simulink model "manul_model_stage15_complete"  (R2025a)
settings: Solver=ode3  StartTime=0.0  StopTime=0.3  FixedStep=Ts_power  RelTol=1e-3
InitFcn:
  | run('D:/PV_MPPT/PV_ESS_MPC_Manul_Reproduction/experiments/stage15_bus_stability_20260814/pvess_stage15_busfix_init.m')
values from neighbouring files (symbols this model uses):
  a_vbat_limit = exp(-2*pi*fc_vbat_limit*Ts_bat_ctrl)    [pvess_stage15_busfix_init.m]    (also in pvess_stage15_busfix_init_pre_cpl_20260817.m; pvess_stage15_busfix_init_pre_gridpi_tuning_20260817.m)
  Ad_mpvc = expm(A_mpvc*Ts_mpc)    [pvess_beginner_init_baseline.m]    (also in pvess_stage15_busfix_init.m; pvess_stage15_busfix_init_pre_cpl_20260817.m; pvess_stage15_busfix_init_pre_engineering_20260816.m; pvess_stage15_busfix_init_pre_gridpi_tuning_20260817.m)
  Bd_mpvc = A_mpvc\((Ad_mpvc-eye(2))*B_mpvc)    [pvess_beginner_init_baseline.m]    (also in pvess_stage15_busfix_init.m; pvess_stage15_busfix_init_pre_cpl_20260817.m; pvess_stage15_busfix_init_pre_engineering_20260816.m; pvess_stage15_busfix_init_pre_gridpi_tuning_20260817.m)
  Cdc = 18e-3    (= 0.018)    [pvess_beginner_init_baseline.m]    (also in pvess_stage15_busfix_init.m; pvess_stage15_busfix_init_pre_cpl_20260817.m; pvess_stage15_busfix_init_pre_engineering_20260816.m; pvess_stage15_busfix_init_pre_gridpi_tuning_20260817.m)
  Cpv = 10e-3    (= 0.01)    [pvess_beginner_init_baseline.m]    (also in pvess_stage15_busfix_init.m; pvess_stage15_busfix_init_pre_cpl_20260817.m; pvess_stage15_busfix_init_pre_engineering_20260816.m; pvess_stage15_busfix_init_pre_gridpi_tuning_20260817.m)
  Db0 = 1 - V_bat_nom/Vdc_ref    (= 0.75)    [pvess_beginner_init_baseline.m]    (also in pvess_stage15_busfix_init.m; pvess_stage15_busfix_init_pre_cpl_20260817.m; pvess_stage15_busfix_init_pre_engineering_20260816.m; pvess_stage15_busfix_init_pre_gridpi_tuning_20260817.m)
  Db_max = 0.95    [pvess_beginner_init_baseline.m]    (also in pvess_stage15_busfix_init.m; pvess_stage15_busfix_init_pre_cpl_20260817.m; pvess_stage15_busfix_init_pre_engineering_20260816.m; pvess_stage15_busfix_init_pre_gridpi_tuning_20260817.m)
  Db_min = 0.05    [pvess_beginner_init_baseline.m]    (also in pvess_stage15_busfix_init.m; pvess_stage15_busfix_init_pre_cpl_20260817.m; pvess_stage15_busfix_init_pre_engineering_20260816.m; pvess_stage15_busfix_init_pre_gridpi_tuning_20260817.m)
  Dcorr_max = Db_max - Db0    (= 0.2)    [pvess_stage15_busfix_init.m]    (also in pvess_stage15_busfix_init_pre_cpl_20260817.m; pvess_stage15_busfix_init_pre_gridpi_tuning_20260817.m)
  Dcorr_min = -0.25    [pvess_stage15_busfix_init.m]    (also in pvess_stage15_busfix_init_pre_cpl_20260817.m; pvess_stage15_busfix_init_pre_gridpi_tuning_20260817.m)
  Dpv0 = 1 - 547/Vdc_ref    (= 0.544166666667)    [pvess_beginner_init_baseline.m]    (also in pvess_stage15_busfix_init.m; pvess_stage15_busfix_init_pre_cpl_20260817.m; pvess_stage15_busfix_init_pre_engineering_20260816.m; pvess_stage15_busfix_init_pre_gridpi_tuning_20260817.m)
  Dpv_curtail_bias = 0.506    [pvess_stage15_busfix_init.m]    (also in pvess_stage15_busfix_init_pre_cpl_20260817.m; pvess_stage15_busfix_init_pre_engineering_20260816.m; pvess_stage15_busfix_init_pre_gridpi_tuning_20260817.m)
  Dpv_max = 0.75    [pvess_beginner_init_baseline.m]    (also in pvess_stage15_busfix_init.m; pvess_stage15_busfix_init_pre_cpl_20260817.m; pvess_stage15_busfix_init_pre_engineering_20260816.m; pvess_stage15_busfix_init_pre_gridpi_tuning_20260817.m)
  Dpv_min = 0.35    [pvess_beginner_init_baseline.m]    (also in pvess_stage15_busfix_init.m; pvess_stage15_busfix_init_pre_cpl_20260817.m; pvess_stage15_busfix_init_pre_engineering_20260816.m; pvess_stage15_busfix_init_pre_gridpi_tuning_20260817.m)
  Dpv_slew_down = -5.0    (= -5)    [pvess_stage15_busfix_init.m]    (also in pvess_stage15_busfix_init_pre_cpl_20260817.m; pvess_stage15_busfix_init_pre_engineering_20260816.m; pvess_stage15_busfix_init_pre_gridpi_tuning_20260817.m)
  Dpv_slew_up = 1.0    (= 1)    [pvess_stage15_busfix_init.m]    (also in pvess_stage15_busfix_init_pre_cpl_20260817.m; pvess_stage15_busfix_init_pre_engineering_20260816.m; pvess_stage15_busfix_init_pre_gridpi_tuning_20260817.m)
  Dpv_step = 2e-4    (= 0.0002)    [pvess_beginner_init_baseline.m]    (also in pvess_stage15_busfix_init.m; pvess_stage15_busfix_init_pre_cpl_20260817.m; pvess_stage15_busfix_init_pre_engineering_20260816.m; pvess_stage15_busfix_init_pre_gridpi_tuning_20260817.m)
  eps_dI = 1e-3    (= 0.001)    [pvess_beginner_init_baseline.m]    (also in pvess_stage15_busfix_init.m; pvess_stage15_busfix_init_pre_cpl_20260817.m; pvess_stage15_busfix_init_pre_engineering_20260816.m; pvess_stage15_busfix_init_pre_gridpi_tuning_20260817.m)
  eps_dV = 1e-3    (= 0.001)    [pvess_beginner_init_baseline.m]    (also in pvess_stage15_busfix_init.m; pvess_stage15_busfix_init_pre_cpl_20260817.m; pvess_stage15_busfix_init_pre_engineering_20260816.m; pvess_stage15_busfix_init_pre_gridpi_tuning_20260817.m)
  eps_inc = 1e-4    (= 0.0001)    [pvess_beginner_init_baseline.m]    (also in pvess_stage15_busfix_init.m; pvess_stage15_busfix_init_pre_cpl_20260817.m; pvess_stage15_busfix_init_pre_engineering_20260816.m; pvess_stage15_busfix_init_pre_gridpi_tuning_20260817.m)
  f_grid = 50    [pvess_beginner_init_baseline.m]    (also in pvess_stage15_busfix_init.m; pvess_stage15_busfix_init_pre_cpl_20260817.m; pvess_stage15_busfix_init_pre_engineering_20260816.m; pvess_stage15_busfix_init_pre_gridpi_tuning_20260817.m)
  freq_threshold = 0.15    [pvess_beginner_init_baseline.m]    (also in pvess_stage15_busfix_init.m; pvess_stage15_busfix_init_pre_cpl_20260817.m; pvess_stage15_busfix_init_pre_engineering_20260816.m; pvess_stage15_busfix_init_pre_gridpi_tuning_20260817.m)
  Iac_rated_lv = S_tr/(sqrt(3)*V_tr_lv)    [pvess_stage15_busfix_init.m]    (also in pvess_stage15_busfix_init_pre_cpl_20260817.m; pvess_stage15_busfix_init_pre_gridpi_tuning_20260817.m)
  Ibat_chg_hw = Ibat_max    (= 1666.66666667)    [pvess_stage15_busfix_init.m]    (also in pvess_stage15_busfix_init_pre_cpl_20260817.m; pvess_stage15_busfix_init_pre_gridpi_tuning_20260817.m)
  Ibat_curtail_release = -0.8*Ibat_max    (= -1333.33333333)    [pvess_stage15_busfix_init.m]    (also in pvess_stage15_busfix_init_pre_cpl_20260817.m; pvess_stage15_busfix_init_pre_engineering_20260816.m; pvess_stage15_busfix_init_pre_gridpi_tuning_20260817.m)
  Ibat_dis_hw = Ibat_max    (= 1666.66666667)    [pvess_stage15_busfix_init.m]    (also in pvess_stage15_busfix_init_pre_cpl_20260817.m; pvess_stage15_busfix_init_pre_gridpi_tuning_20260817.m)
  Ibat_max = P_bat_rated/V_bat_nom    (= 1666.66666667)    [pvess_beginner_init_baseline.m]    (also in pvess_stage15_busfix_init.m; pvess_stage15_busfix_init_pre_cpl_20260817.m; pvess_stage15_busfix_init_pre_engineering_20260816.m; pvess_stage15_busfix_init_pre_gridpi_tuning_20260817.m)
  Ilim_eps = 1    [pvess_stage15_busfix_init.m]    (also in pvess_stage15_busfix_init_pre_cpl_20260817.m; pvess_stage15_busfix_init_pre_gridpi_tuning_20260817.m)
  K_bat_sign = 1    [pvess_beginner_init_baseline.m]    (also in pvess_stage15_busfix_init.m; pvess_stage15_busfix_init_pre_cpl_20260817.m; pvess_stage15_busfix_init_pre_engineering_20260816.m; pvess_stage15_busfix_init_pre_gridpi_tuning_20260817.m)
  K_grid_sign = -1    [pvess_beginner_init_baseline.m]    (also in pvess_stage15_busfix_init.m; pvess_stage15_busfix_init_pre_cpl_20260817.m; pvess_stage15_busfix_init_pre_engineering_20260816.m; pvess_stage15_busfix_init_pre_gridpi_tuning_20260817.m)
  Ki_dc = 3.40748e5    (= 340748)    [pvess_beginner_init_baseline.m]    (also in pvess_stage15_busfix_init.m = 2131834.55064; pvess_stage15_busfix_init_pre_cpl_20260817.m; pvess_stage15_busfix_init_pre_engineering_20260816.m; pvess_stage15_busfix_init_pre_gridpi_tuning_20260817.m)
  Kii_bat = 0.150    (= 0.15)    [pvess_beginner_init_baseline.m]    (also in pvess_stage15_busfix_init.m = 0.05; pvess_stage15_busfix_init_pre_cpl_20260817.m = 0.05; pvess_stage15_busfix_init_pre_engineering_20260816.m = 0.05; pvess_stage15_busfix_init_pre_gridpi_tuning_20260817.m = 0.05)
  Kiv_bat = 650    [pvess_beginner_init_baseline.m]    (also in pvess_stage15_busfix_init.m; pvess_stage15_busfix_init_pre_cpl_20260817.m; pvess_stage15_busfix_init_pre_engineering_20260816.m; pvess_stage15_busfix_init_pre_gridpi_tuning_20260817.m)
  Kp_dc = 3836.125    [pvess_beginner_init_baseline.m]    (also in pvess_stage15_busfix_init.m = 2*zeta_dc*(2*pi*f_bw_dc)*Cdc*Vdc_ref; pvess_stage15_busfix_init_pre_cpl_20260817.m; pvess_stage15_busfix_init_pre_engineering_20260816.m; pvess_stage15_busfix_init_pre_gridpi_tuning_20260817.m)
  Kp_pv_curtail = 5e-5    (= 5e-05)    [pvess_stage15_busfix_init.m]    (also in pvess_stage15_busfix_init_pre_cpl_20260817.m; pvess_stage15_busfix_init_pre_engineering_20260816.m; pvess_stage15_busfix_init_pre_gridpi_tuning_20260817.m)
  Kpi_bat = 100e-3    (= 0.1)    [pvess_beginner_init_baseline.m]    (also in pvess_stage15_busfix_init.m = 0.005; pvess_stage15_busfix_init_pre_cpl_20260817.m = 0.005; pvess_stage15_busfix_init_pre_engineering_20260816.m = 0.005; pvess_stage15_busfix_init_pre_gridpi_tuning_20260817.m = 0.005)
  Kpv_bat = 4    [pvess_beginner_init_baseline.m]    (also in pvess_stage15_busfix_init.m; pvess_stage15_busfix_init_pre_cpl_20260817.m; pvess_stage15_busfix_init_pre_engineering_20260816.m; pvess_stage15_busfix_init_pre_gridpi_tuning_20260817.m)
  Kt_bat = 143    [pvess_stage15_busfix_init.m]    (also in pvess_stage15_busfix_init_pre_cpl_20260817.m; pvess_stage15_busfix_init_pre_gridpi_tuning_20260817.m)
  lambda_mppc = 0.001    [pvess_beginner_init_baseline.m]    (also in pvess_stage15_busfix_init.m; pvess_stage15_busfix_init_pre_cpl_20260817.m; pvess_stage15_busfix_init_pre_engineering_20260816.m; pvess_stage15_busfix_init_pre_gridpi_tuning_20260817.m)
  lambda_mpvc = 3e-6    (= 3e-06)    [pvess_beginner_init_baseline.m]    (also in pvess_stage15_busfix_init.m; pvess_stage15_busfix_init_pre_cpl_20260817.m; pvess_stage15_busfix_init_pre_engineering_20260816.m; pvess_stage15_busfix_init_pre_gridpi_tuning_20260817.m)
  Lbat = 11.25e-3    (= 0.01125)    [pvess_beginner_init_baseline.m]    (also in pvess_stage15_busfix_init.m = 0.0005; pvess_stage15_busfix_init_pre_cpl_20260817.m = 0.0005; pvess_stage15_busfix_init_pre_engineering_20260816.m = 0.0005; pvess_stage15_busfix_init_pre_gridpi_tuning_20260817.m = 0.0005)
  Lf = 0.6e-3    (= 0.0006)    [pvess_beginner_init_baseline.m]    (also in pvess_stage15_busfix_init.m; pvess_stage15_busfix_init_pre_cpl_20260817.m; pvess_stage15_busfix_init_pre_engineering_20260816.m; pvess_stage15_busfix_init_pre_gridpi_tuning_20260817.m)
  Lpv = 0.8e-3    (= 0.0008)    [pvess_beginner_init_baseline.m]    (also in pvess_stage15_busfix_init.m; pvess_stage15_busfix_init_pre_cpl_20260817.m; pvess_stage15_busfix_init_pre_engineering_20260816.m; pvess_stage15_busfix_init_pre_gridpi_tuning_20260817.m)
  m_var = 4e6    (= 4000000)    [pvess_beginner_init_baseline.m]    (also in pvess_stage15_busfix_init.m; pvess_stage15_busfix_init_pre_cpl_20260817.m; pvess_stage15_busfix_init_pre_engineering_20260816.m; pvess_stage15_busfix_init_pre_gridpi_tuning_20260817.m)
  N_ems_fast_avg = 100    [pvess_beginner_init_baseline.m]    (also in pvess_stage15_busfix_init.m; pvess_stage15_busfix_init_pre_cpl_20260817.m; pvess_stage15_busfix_init_pre_engineering_20260816.m; pvess_stage15_busfix_init_pre_gridpi_tuning_20260817.m)
  omega_grid = 2*pi*f_grid    (= 314.159265359)    [pvess_beginner_init_baseline.m]    (also in pvess_stage15_busfix_init.m; pvess_stage15_busfix_init_pre_cpl_20260817.m; pvess_stage15_busfix_init_pre_engineering_20260816.m; pvess_stage15_busfix_init_pre_gridpi_tuning_20260817.m)
  P_base_mpc = 2e6    (= 2000000)    [pvess_beginner_init_baseline.m]    (also in pvess_stage15_busfix_init.m; pvess_stage15_busfix_init_pre_cpl_20260817.m; pvess_stage15_busfix_init_pre_engineering_20260816.m; pvess_stage15_busfix_init_pre_gridpi_tuning_20260817.m)
  Pbat_chg_max = P_bat_rated    (= 500000)    [pvess_stage15_busfix_init.m]    (also in pvess_stage15_busfix_init_pre_cpl_20260817.m; pvess_stage15_busfix_init_pre_gridpi_tuning_20260817.m)
  Pbat_dis_max = P_bat_rated    (= 500000)    [pvess_stage15_busfix_init.m]    (also in pvess_stage15_busfix_init_pre_cpl_20260817.m; pvess_stage15_busfix_init_pre_gridpi_tuning_20260817.m)
  Pdc_cpl_eps = 100    [pvess_stage15_busfix_init.m]    (also in pvess_stage15_busfix_init_pre_gridpi_tuning_20260817.m)
  phase_threshold = 0.99863    [pvess_beginner_init_baseline.m]    (also in pvess_stage15_busfix_init.m; pvess_stage15_busfix_init_pre_cpl_20260817.m; pvess_stage15_busfix_init_pre_engineering_20260816.m; pvess_stage15_busfix_init_pre_gridpi_tuning_20260817.m)
  PQLimit_eps = 1e3    (= 1000)    [pvess_stage15_busfix_init.m]    (also in pvess_stage15_busfix_init_pre_cpl_20260817.m; pvess_stage15_busfix_init_pre_gridpi_tuning_20260817.m)
  Pref_max = 2.2e6    (= 2200000)    [pvess_beginner_init_baseline.m]    (also in pvess_stage15_busfix_init.m; pvess_stage15_busfix_init_pre_cpl_20260817.m; pvess_stage15_busfix_init_pre_engineering_20260816.m; pvess_stage15_busfix_init_pre_gridpi_tuning_20260817.m)
  Pref_min = -2.2e6    (= -2200000)    [pvess_beginner_init_baseline.m]    (also in pvess_stage15_busfix_init.m; pvess_stage15_busfix_init_pre_cpl_20260817.m; pvess_stage15_busfix_init_pre_engineering_20260816.m; pvess_stage15_busfix_init_pre_gridpi_tuning_20260817.m)
  Q_base_mpc = 1e6    (= 1000000)    [pvess_beginner_init_baseline.m]    (also in pvess_stage15_busfix_init.m; pvess_stage15_busfix_init_pre_cpl_20260817.m; pvess_stage15_busfix_init_pre_engineering_20260816.m; pvess_stage15_busfix_init_pre_gridpi_tuning_20260817.m)
  Q_bat_Ah = 1300    [pvess_beginner_init_baseline.m]    (also in pvess_stage15_busfix_init.m; pvess_stage15_busfix_init_pre_cpl_20260817.m; pvess_stage15_busfix_init_pre_engineering_20260816.m; pvess_stage15_busfix_init_pre_gridpi_tuning_20260817.m)
  R_bat_internal = 0.02    [pvess_beginner_init_baseline.m]    (also in pvess_stage15_busfix_init.m; pvess_stage15_busfix_init_pre_cpl_20260817.m; pvess_stage15_busfix_init_pre_engineering_20260816.m; pvess_stage15_busfix_init_pre_gridpi_tuning_20260817.m)
  Rdc_cpl_min = 0.2    [pvess_stage15_busfix_init.m]    (also in pvess_stage15_busfix_init_pre_gridpi_tuning_20260817.m)
  Rdc_cpl_off = 1e6    (= 1000000)    [pvess_stage15_busfix_init.m]    (also in pvess_stage15_busfix_init_pre_gridpi_tuning_20260817.m)
  Rf = 0.019    [pvess_beginner_init_baseline.m]    (also in pvess_stage15_busfix_init.m; pvess_stage15_busfix_init_pre_cpl_20260817.m; pvess_stage15_busfix_init_pre_engineering_20260816.m; pvess_stage15_busfix_init_pre_gridpi_tuning_20260817.m)
  RLbat = 2e-3    (= 0.002)    [pvess_beginner_init_baseline.m]    (also in pvess_stage15_busfix_init.m; pvess_stage15_busfix_init_pre_cpl_20260817.m; pvess_stage15_busfix_init_pre_engineering_20260816.m; pvess_stage15_busfix_init_pre_gridpi_tuning_20260817.m)
  RLpv = 2e-3    (= 0.002)    [pvess_beginner_init_baseline.m]    (also in pvess_stage15_busfix_init.m; pvess_stage15_busfix_init_pre_cpl_20260817.m; pvess_stage15_busfix_init_pre_engineering_20260816.m; pvess_stage15_busfix_init_pre_gridpi_tuning_20260817.m)
  S_tr = 2.5e6    (= 2500000)    [pvess_beginner_init_baseline.m]    (also in pvess_stage15_busfix_init.m; pvess_stage15_busfix_init_pre_cpl_20260817.m; pvess_stage15_busfix_init_pre_engineering_20260816.m; pvess_stage15_busfix_init_pre_gridpi_tuning_20260817.m)
  SOC0 = 50    [pvess_beginner_init_baseline.m]    (also in pvess_stage15_busfix_init.m; pvess_stage15_busfix_init_pre_cpl_20260817.m; pvess_stage15_busfix_init_pre_engineering_20260816.m; pvess_stage15_busfix_init_pre_gridpi_tuning_20260817.m)
  SOC_chg_bp = [0 85 90 100]    [pvess_stage15_busfix_init.m]    (also in pvess_stage15_busfix_init_pre_cpl_20260817.m; pvess_stage15_busfix_init_pre_gridpi_tuning_20260817.m)
  SOC_chg_k = [1  1  0   0]    [pvess_stage15_busfix_init.m]    (also in pvess_stage15_busfix_init_pre_cpl_20260817.m; pvess_stage15_busfix_init_pre_gridpi_tuning_20260817.m)
  SOC_dis_bp = [0 10 15 100]    [pvess_stage15_busfix_init.m]    (also in pvess_stage15_busfix_init_pre_cpl_20260817.m; pvess_stage15_busfix_init_pre_gridpi_tuning_20260817.m)
  SOC_dis_k = [0  0  1   1]    [pvess_stage15_busfix_init.m]    (also in pvess_stage15_busfix_init_pre_cpl_20260817.m; pvess_stage15_busfix_init_pre_gridpi_tuning_20260817.m)
  SOC_max = 90    [pvess_beginner_init_baseline.m]    (also in pvess_stage15_busfix_init.m; pvess_stage15_busfix_init_pre_cpl_20260817.m; pvess_stage15_busfix_init_pre_engineering_20260816.m; pvess_stage15_busfix_init_pre_gridpi_tuning_20260817.m)
  SOC_min = 10    [pvess_beginner_init_baseline.m]    (also in pvess_stage15_busfix_init.m; pvess_stage15_busfix_init_pre_cpl_20260817.m; pvess_stage15_busfix_init_pre_engineering_20260816.m; pvess_stage15_busfix_init_pre_gridpi_tuning_20260817.m)
  sync_hold = 0.1    [pvess_beginner_init_baseline.m]    (also in pvess_stage15_busfix_init.m; pvess_stage15_busfix_init_pre_cpl_20260817.m; pvess_stage15_busfix_init_pre_engineering_20260816.m; pvess_stage15_busfix_init_pre_gridpi_tuning_20260817.m)
  T_ac_step = 0.2    [pvess_beginner_init_baseline.m]    (also in pvess_stage15_busfix_init.m = 0.5; pvess_stage15_busfix_init_pre_cpl_20260817.m = 0.5; pvess_stage15_busfix_init_pre_engineering_20260816.m = 0.5; pvess_stage15_busfix_init_pre_gridpi_tuning_20260817.m = 0.5)
  T_grid_connect = 1.6    [pvess_beginner_init_baseline.m]    (also in pvess_stage15_busfix_init.m; pvess_stage15_busfix_init_pre_cpl_20260817.m; pvess_stage15_busfix_init_pre_engineering_20260816.m; pvess_stage15_busfix_init_pre_gridpi_tuning_20260817.m)
  T_grid_dip = 3.5    [pvess_beginner_init_baseline.m]    (also in pvess_stage15_busfix_init.m; pvess_stage15_busfix_init_pre_cpl_20260817.m; pvess_stage15_busfix_init_pre_engineering_20260816.m; pvess_stage15_busfix_init_pre_gridpi_tuning_20260817.m)
  T_sync = 1.4    [pvess_beginner_init_baseline.m]    (also in pvess_stage15_busfix_init.m; pvess_stage15_busfix_init_pre_cpl_20260817.m; pvess_stage15_busfix_init_pre_engineering_20260816.m; pvess_stage15_busfix_init_pre_gridpi_tuning_20260817.m)
  Ts_bat_ctrl = 100e-6    (= 0.0001)    [pvess_beginner_init_baseline.m]    (also in pvess_stage15_busfix_init.m; pvess_stage15_busfix_init_pre_cpl_20260817.m; pvess_stage15_busfix_init_pre_engineering_20260816.m; pvess_stage15_busfix_init_pre_gridpi_tuning_20260817.m)
  Ts_cpl = 1/20e3    (= 5e-05)    [pvess_stage15_busfix_init.m]    (also in pvess_stage15_busfix_init_pre_gridpi_tuning_20260817.m)
  Ts_ems = 1e-3    (= 0.001)    [pvess_beginner_init_baseline.m]    (also in pvess_stage15_busfix_init.m; pvess_stage15_busfix_init_pre_cpl_20260817.m; pvess_stage15_busfix_init_pre_engineering_20260816.m; pvess_stage15_busfix_init_pre_gridpi_tuning_20260817.m)
  Ts_mpc = 1/20e3    (= 5e-05)    [pvess_beginner_init_baseline.m]    (also in pvess_stage15_busfix_init.m; pvess_stage15_busfix_init_pre_cpl_20260817.m; pvess_stage15_busfix_init_pre_engineering_20260816.m; pvess_stage15_busfix_init_pre_gridpi_tuning_20260817.m)
  Ts_mppt = 1e-3    (= 0.001)    [pvess_beginner_init_baseline.m]    (also in pvess_stage15_busfix_init.m; pvess_stage15_busfix_init_pre_cpl_20260817.m; pvess_stage15_busfix_init_pre_engineering_20260816.m; pvess_stage15_busfix_init_pre_gridpi_tuning_20260817.m)
  Ts_power = 2e-6    (= 2e-06)    [pvess_beginner_init_baseline.m]    (also in pvess_stage15_busfix_init.m; pvess_stage15_busfix_init_pre_cpl_20260817.m; pvess_stage15_busfix_init_pre_engineering_20260816.m; pvess_stage15_busfix_init_pre_gridpi_tuning_20260817.m)
  Ts_soc = 1e-4    (= 0.0001)    [pvess_beginner_init_baseline.m]    (also in pvess_stage15_busfix_init.m; pvess_stage15_busfix_init_pre_cpl_20260817.m; pvess_stage15_busfix_init_pre_engineering_20260816.m; pvess_stage15_busfix_init_pre_gridpi_tuning_20260817.m)
  V_bat_nom = 300    [pvess_beginner_init_baseline.m]    (also in pvess_stage15_busfix_init.m; pvess_stage15_busfix_init_pre_cpl_20260817.m; pvess_stage15_busfix_init_pre_engineering_20260816.m; pvess_stage15_busfix_init_pre_gridpi_tuning_20260817.m)
  V_tr_hv = 25e3    (= 25000)    [pvess_beginner_init_baseline.m]    (also in pvess_stage15_busfix_init.m; pvess_stage15_busfix_init_pre_cpl_20260817.m; pvess_stage15_busfix_init_pre_engineering_20260816.m; pvess_stage15_busfix_init_pre_gridpi_tuning_20260817.m)
  V_tr_lv = Vac_ll    (= 690)    [pvess_beginner_init_baseline.m]    (also in pvess_stage15_busfix_init.m; pvess_stage15_busfix_init_pre_cpl_20260817.m; pvess_stage15_busfix_init_pre_engineering_20260816.m; pvess_stage15_busfix_init_pre_gridpi_tuning_20260817.m)
  Vac_phase_peak = sqrt(2)*Vac_ll/sqrt(3)    [pvess_beginner_init_baseline.m]    (also in pvess_stage15_busfix_init.m; pvess_stage15_busfix_init_pre_cpl_20260817.m; pvess_stage15_busfix_init_pre_engineering_20260816.m; pvess_stage15_busfix_init_pre_gridpi_tuning_20260817.m)
  Vbat_div_floor = 270    [pvess_stage15_busfix_init.m]    (also in pvess_stage15_busfix_init_pre_cpl_20260817.m; pvess_stage15_busfix_init_pre_gridpi_tuning_20260817.m)
  Vdc_cpl_floor = 0.70*Vdc_ref    (= 840)    [pvess_stage15_busfix_init.m]    (also in pvess_stage15_busfix_init_pre_gridpi_tuning_20260817.m)
  Vdc_curtail_off = 1185    [pvess_stage15_busfix_init.m]    (also in pvess_stage15_busfix_init_pre_cpl_20260817.m; pvess_stage15_busfix_init_pre_engineering_20260816.m; pvess_stage15_busfix_init_pre_gridpi_tuning_20260817.m)
  Vdc_curtail_on = 1220    [pvess_stage15_busfix_init.m]    (also in pvess_stage15_busfix_init_pre_cpl_20260817.m; pvess_stage15_busfix_init_pre_engineering_20260816.m; pvess_stage15_busfix_init_pre_gridpi_tuning_20260817.m)
  Vdc_ref = 1200    [pvess_beginner_init_baseline.m]    (also in pvess_stage15_busfix_init.m; pvess_stage15_busfix_init_pre_cpl_20260817.m; pvess_stage15_busfix_init_pre_engineering_20260816.m; pvess_stage15_busfix_init_pre_gridpi_tuning_20260817.m)
  Vf_diode = 1.0    (= 1)    [pvess_beginner_init_baseline.m]    (also in pvess_stage15_busfix_init.m; pvess_stage15_busfix_init_pre_cpl_20260817.m; pvess_stage15_busfix_init_pre_engineering_20260816.m; pvess_stage15_busfix_init_pre_gridpi_tuning_20260817.m)
  Vgrid_limit_floor = 0.1*V_tr_lv    (= 69)    [pvess_stage15_busfix_init.m]    (also in pvess_stage15_busfix_init_pre_cpl_20260817.m; pvess_stage15_busfix_init_pre_gridpi_tuning_20260817.m)
  Vpv0 = 547    [pvess_beginner_init_baseline.m]    (also in pvess_stage15_busfix_init.m; pvess_stage15_busfix_init_pre_cpl_20260817.m; pvess_stage15_busfix_init_pre_engineering_20260816.m; pvess_stage15_busfix_init_pre_gridpi_tuning_20260817.m)
  Vsync_threshold = 10    [pvess_beginner_init_baseline.m]    (also in pvess_stage15_busfix_init.m; pvess_stage15_busfix_init_pre_cpl_20260817.m; pvess_stage15_busfix_init_pre_engineering_20260816.m; pvess_stage15_busfix_init_pre_gridpi_tuning_20260817.m)
undefined symbols (not defined in the file or in its folder): DiscIntNeverNeededParam, dspblkCoreblockFVToolHelper, gcbh, Ion, Kt_dc, Lithium
libraries: simulink x14, dspstat3 x10, spsBreakerLib x5, spsCurrentMeasurementLib x4, slpidlib x3, spsThreePhaseVIMeasurementLib x3, eeRmsMeasurement x3, spsThreePhaseParallelRLCLoadLib x3, spsThreePhaseBreakerLib x3, spsParallelRLCBranchLib x2, spsVariableResistorLib x2, spsThreePhaseSeriesRLCBranchLib x2
(part 2 of 3)

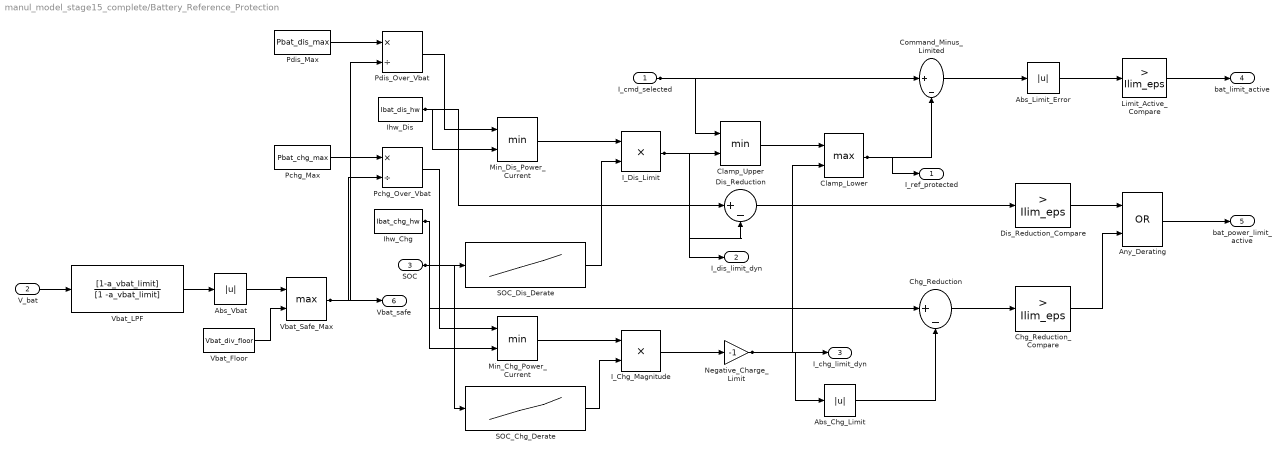
== system manul_model_stage15_complete/Battery_Reference_Protection ==
  I_cmd_selected : Inport
  V_bat : Inport  Port=2
  SOC : Inport  Port=3
  Abs_Chg_Limit : Abs  SaturateOnIntegerOverflow=off
  Abs_Limit_Error : Abs  SaturateOnIntegerOverflow=off
  Abs_Vbat : Abs  SaturateOnIntegerOverflow=off
  Any_Derating : Logic  Operator=OR  AllPortsSameDT=off  OutDataTypeStr=boolean
  Chg_Reduction : Sum  Inputs=|+-
  Chg_Reduction_Compare : simulink/Logic and Bit Operations/Compare To Constant  relop=>  const=Ilim_eps  OutDataTypeStr=boolean
  Clamp_Lower : MinMax  Function=max  Inputs=2
  Clamp_Upper : MinMax  Inputs=2
  Command_Minus_Limited : Sum  Inputs=|+-
  Dis_Reduction : Sum  Inputs=|+-
  Dis_Reduction_Compare : simulink/Logic and Bit Operations/Compare To Constant  relop=>  const=Ilim_eps  OutDataTypeStr=boolean
  I_Chg_Magnitude : Product  Inputs=**
  I_Dis_Limit : Product  Inputs=**
  Ihw_Chg : Constant  Value=Ibat_chg_hw
  Ihw_Dis : Constant  Value=Ibat_dis_hw
  Limit_Active_Compare : simulink/Logic and Bit Operations/Compare To Constant  relop=>  const=Ilim_eps  OutDataTypeStr=boolean
  Min_Chg_Power_Current : MinMax  Inputs=2
  Min_Dis_Power_Current : MinMax  Inputs=2
  Negative_Charge_Limit : Gain  Gain=-1
  Pchg_Max : Constant  Value=Pbat_chg_max
  Pchg_Over_Vbat : Product  Inputs=*/
  Pdis_Max : Constant  Value=Pbat_dis_max
  Pdis_Over_Vbat : Product  Inputs=*/
  SOC_Chg_Derate : Lookup_n-D  NumberOfTableDimensions=1  BreakpointsForDimension1=SOC_chg_bp  Table=SOC_chg_k  ExtrapMethod=Clip  InternalRulePriority=Speed  RndMeth=Simplest
  SOC_Dis_Derate : Lookup_n-D  NumberOfTableDimensions=1  BreakpointsForDimension1=SOC_dis_bp  Table=SOC_dis_k  ExtrapMethod=Clip  InternalRulePriority=Speed  RndMeth=Simplest
  Vbat_Floor : Constant  Value=Vbat_div_floor
  Vbat_LPF : DiscreteTransferFcn  Numerator=[1-a_vbat_limit]  Denominator=[1 -a_vbat_limit]  InitialStates=V_bat_nom  SampleTime=Ts_bat_ctrl
  Vbat_Safe_Max : MinMax  Function=max  Inputs=2
  I_ref_protected : Outport
  I_dis_limit_dyn : Outport  Port=2
  I_chg_limit_dyn : Outport  Port=3
  bat_limit_active : Outport  Port=4
  bat_power_limit_active : Outport  Port=5
  Vbat_safe : Outport  Port=6
  wires:
  Abs_Vbat/1 -> Vbat_Safe_Max/1
  Vbat_Safe_Max/1 -> Pchg_Over_Vbat/2, Vbat_safe/1, Pdis_Over_Vbat/2
  I_cmd_selected/1 -> Command_Minus_Limited/1, Clamp_Upper/1
  SOC/1 -> SOC_Dis_Derate/1, SOC_Chg_Derate/1
  Vbat_LPF/1 -> Abs_Vbat/1
  Abs_Limit_Error/1 -> Limit_Active_Compare/1
  V_bat/1 -> Vbat_LPF/1
  Pchg_Over_Vbat/1 -> Min_Chg_Power_Current/1
  Pchg_Max/1 -> Pchg_Over_Vbat/1
  Negative_Charge_Limit/1 -> Clamp_Lower/2, I_chg_limit_dyn/1, Abs_Chg_Limit/1
  Min_Dis_Power_Current/1 -> I_Dis_Limit/1
  Vbat_Floor/1 -> Vbat_Safe_Max/2
  Pdis_Max/1 -> Pdis_Over_Vbat/1
  Pdis_Over_Vbat/1 -> Min_Dis_Power_Current/1
  I_Chg_Magnitude/1 -> Negative_Charge_Limit/1
  I_Dis_Limit/1 -> Dis_Reduction/2, Clamp_Upper/2, I_dis_limit_dyn/1
  Ihw_Dis/1 -> Dis_Reduction/1, Min_Dis_Power_Current/2
  Min_Chg_Power_Current/1 -> I_Chg_Magnitude/1
  Ihw_Chg/1 -> Chg_Reduction/1, Min_Chg_Power_Current/2
  SOC_Dis_Derate/1 -> I_Dis_Limit/2
  SOC_Chg_Derate/1 -> I_Chg_Magnitude/2
  Dis_Reduction_Compare/1 -> Any_Derating/1
  Clamp_Upper/1 -> Clamp_Lower/1
  Command_Minus_Limited/1 -> Abs_Limit_Error/1
  Dis_Reduction/1 -> Dis_Reduction_Compare/1
  Clamp_Lower/1 -> Command_Minus_Limited/2, I_ref_protected/1
  Abs_Chg_Limit/1 -> Chg_Reduction/2
  Any_Derating/1 -> bat_power_limit_active/1
  Chg_Reduction/1 -> Chg_Reduction_Compare/1
  Chg_Reduction_Compare/1 -> Any_Derating/2
  Limit_Active_Compare/1 -> bat_limit_active/1

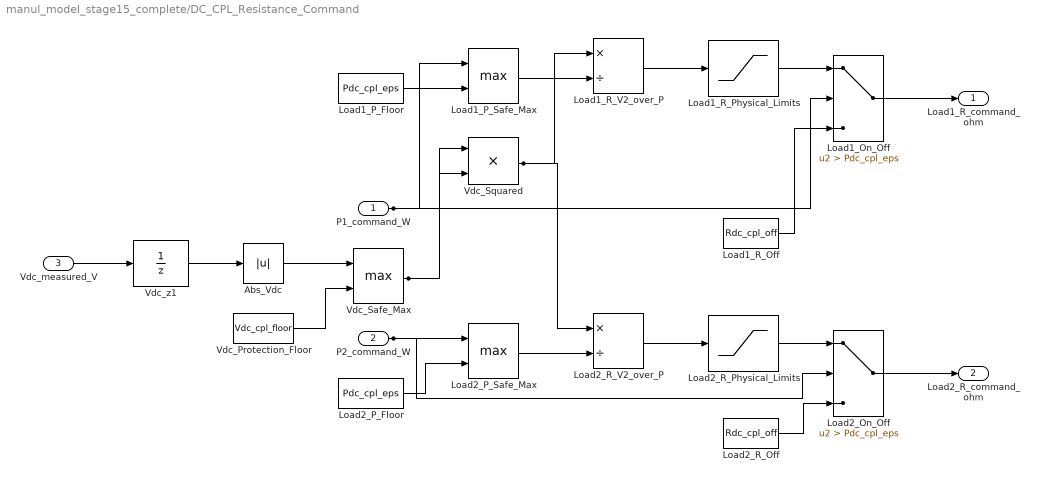
== system manul_model_stage15_complete/DC_CPL_Resistance_Command ==
  P1_command_W : Inport
  P2_command_W : Inport  Port=2
  Vdc_measured_V : Inport  Port=3
  Abs_Vdc : Abs  SaturateOnIntegerOverflow=off
  Load1_On_Off : Switch  Criteria=u2 > Threshold  Threshold=Pdc_cpl_eps  SaturateOnIntegerOverflow=off  InputSameDT=off
  Load1_P_Floor : Constant  Value=Pdc_cpl_eps
  Load1_P_Safe_Max : MinMax  Function=max  Inputs=2
  Load1_R_Off : Constant  Value=Rdc_cpl_off
  Load1_R_Physical_Limits : Saturate  UpperLimit=Rdc_cpl_off  LowerLimit=Rdc_cpl_min
  Load1_R_V2_over_P : Product  Inputs=*/
  Load2_On_Off : Switch  Criteria=u2 > Threshold  Threshold=Pdc_cpl_eps  SaturateOnIntegerOverflow=off  InputSameDT=off
  Load2_P_Floor : Constant  Value=Pdc_cpl_eps
  Load2_P_Safe_Max : MinMax  Function=max  Inputs=2
  Load2_R_Off : Constant  Value=Rdc_cpl_off
  Load2_R_Physical_Limits : Saturate  UpperLimit=Rdc_cpl_off  LowerLimit=Rdc_cpl_min
  Load2_R_V2_over_P : Product  Inputs=*/
  Vdc_Protection_Floor : Constant  Value=Vdc_cpl_floor
  Vdc_Safe_Max : MinMax  Function=max  Inputs=2
  Vdc_Squared : Product  Inputs=**
  Vdc_z1 : UnitDelay  InitialCondition=Vdc_ref  SampleTime=Ts_cpl  HasFrameUpgradeWarning=on
  Load1_R_command_ohm : Outport
  Load2_R_command_ohm : Outport  Port=2
  wires:
  P2_command_W/1 -> Load2_On_Off/2, Load2_P_Safe_Max/1
  P1_command_W/1 -> Load1_On_Off/2, Load1_P_Safe_Max/1
  Load1_P_Floor/1 -> Load1_P_Safe_Max/2
  Load1_R_Physical_Limits/1 -> Load1_On_Off/1
  Abs_Vdc/1 -> Vdc_Safe_Max/1
  Load1_On_Off/1 -> Load1_R_command_ohm/1
  Load1_R_Off/1 -> Load1_On_Off/3
  Vdc_measured_V/1 -> Vdc_z1/1
  Vdc_z1/1 -> Abs_Vdc/1
  Vdc_Safe_Max/1 -> Vdc_Squared/1, Vdc_Squared/2
  Vdc_Squared/1 -> Load1_R_V2_over_P/1, Load2_R_V2_over_P/1
  Vdc_Protection_Floor/1 -> Vdc_Safe_Max/2
  Load2_P_Floor/1 -> Load2_P_Safe_Max/2
  Load1_P_Safe_Max/1 -> Load1_R_V2_over_P/2
  Load2_P_Safe_Max/1 -> Load2_R_V2_over_P/2
  Load1_R_V2_over_P/1 -> Load1_R_Physical_Limits/1
  Load2_R_V2_over_P/1 -> Load2_R_Physical_Limits/1
  Load2_R_Physical_Limits/1 -> Load2_On_Off/1
  Load2_On_Off/1 -> Load2_R_command_ohm/1
  Load2_R_Off/1 -> Load2_On_Off/3

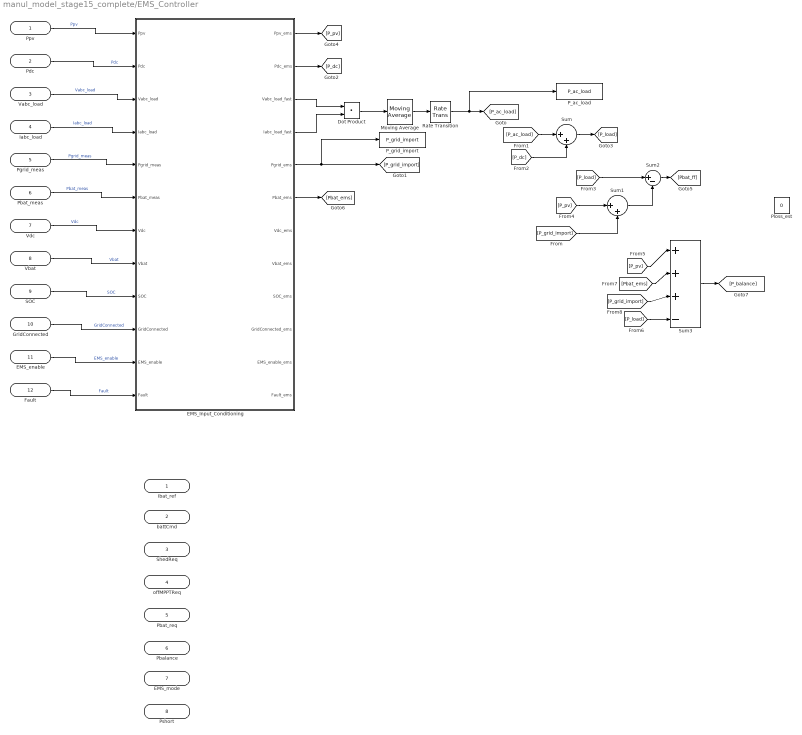
== system manul_model_stage15_complete/EMS_Controller ==
  Ppv : Inport  OutDataTypeStr=double  PortDimensions=1  SampleTime=Ts_power
  Pdc : Inport  Port=2  OutDataTypeStr=double  PortDimensions=1  SampleTime=Ts_power
  Vabc_load : Inport  Port=3  OutDataTypeStr=double  PortDimensions=3  SampleTime=Ts_mpc
  Iabc_load : Inport  Port=4  OutDataTypeStr=double  PortDimensions=3  SampleTime=Ts_mpc
  Pgrid_meas : Inport  Port=5  OutDataTypeStr=double  PortDimensions=1  SampleTime=Ts_mpc
  Pbat_meas : Inport  Port=6  OutDataTypeStr=double  PortDimensions=1  SampleTime=Ts_power
  Vdc : Inport  Port=7  OutDataTypeStr=double  PortDimensions=1  SampleTime=Ts_power
  Vbat : Inport  Port=8  OutDataTypeStr=double  PortDimensions=1  SampleTime=Ts_power
  SOC : Inport  Port=9  OutDataTypeStr=double  PortDimensions=1  SampleTime=Ts_soc
  GridConnected : Inport  Port=10  OutDataTypeStr=boolean  PortDimensions=1
  EMS_enable : Inport  Port=11  OutDataTypeStr=boolean  PortDimensions=1
  Fault : Inport  Port=12  OutDataTypeStr=boolean  PortDimensions=1
  Dot Product : DotProduct  OutDataTypeStr=Inherit: Inherit via internal rule
  EMS_Input_Conditioning : Subsystem
  Moving Average : dspstat3/Moving Average  Method=Sliding window  ForgettingFactorPort=off  SpecifyWindowLength=on  WindowLength=20  OverlapLength=19  AllowArbitraryInputLength=off  ForgettingFactor=0.9  SimulateUsing=Interpreted execution
  P_ac_load : ToWorkspace  VariableName=P_ac_load  SaveFormat=Timeseries  SampleTime=-1
  P_grid_import : ToWorkspace  VariableName=P_grid_import  SaveFormat=Timeseries  SampleTime=-1
  Ploss_est : Constant  Value=0
  Rate Transition : RateTransition  OutPortSampleTime=Ts_ems
  Sum : Sum  Inputs=|++
  Sum1 : Sum  Inputs=|++
  Sum2 : Sum  Inputs=|+-
  Sum3 : Sum  Inputs=|+++-
  Ibat_ref : Outport  OutDataTypeStr=double  PortDimensions=1
  battCmd : Outport  Port=2  OutDataTypeStr=int8  PortDimensions=1
  ShedReq : Outport  Port=3  OutDataTypeStr=boolean  PortDimensions=1
  offMPPTReq : Outport  Port=4  OutDataTypeStr=boolean  PortDimensions=1
  Pbat_req : Outport  Port=5  OutDataTypeStr=double  PortDimensions=1
  Pbalance : Outport  Port=6  OutDataTypeStr=double  PortDimensions=1
  EMS_mode : Outport  Port=7  OutDataTypeStr=int8  PortDimensions=1
  Pshort : Outport  Port=8  OutDataTypeStr=double  PortDimensions=1
  wires:
  Ppv/1 -> EMS_Input_Conditioning/1(Ppv)  "Ppv"
  Pdc/1 -> EMS_Input_Conditioning/2(Pdc)  "Pdc"
  Vabc_load/1 -> EMS_Input_Conditioning/3(Vabc_load)  "Vabc_load"
  Iabc_load/1 -> EMS_Input_Conditioning/4(Iabc_load)  "Iabc_load"
  Pgrid_meas/1 -> EMS_Input_Conditioning/5(Pgrid_meas)  "Pgrid_meas"
  Pbat_meas/1 -> EMS_Input_Conditioning/6(Pbat_meas)  "Pbat_meas"
  Vdc/1 -> EMS_Input_Conditioning/7(Vdc)  "Vdc"
  Vbat/1 -> EMS_Input_Conditioning/8(Vbat)  "Vbat"
  SOC/1 -> EMS_Input_Conditioning/9(SOC)  "SOC"
  GridConnected/1 -> EMS_Input_Conditioning/10(GridConnected)  "GridConnected"
  EMS_enable/1 -> EMS_Input_Conditioning/11(EMS_enable)  "EMS_enable"
  Fault/1 -> EMS_Input_Conditioning/12(Fault)  "Fault"
  EMS_Input_Conditioning/3(Vabc_load_fast) -> Dot Product/1
  EMS_Input_Conditioning/4(Iabc_load_fast) -> Dot Product/2
  Dot Product/1 -> Moving Average/1
  Moving Average/1 -> Rate Transition/1
  Rate Transition/1 -> P_ac_load/1, [P_ac_load]
  EMS_Input_Conditioning/5(Pgrid_ems) -> P_grid_import/1, [P_grid_import]
  EMS_Input_Conditioning/2(Pdc_ems) -> [P_dc]
  [P_ac_load] -> Sum/1
  [P_dc] -> Sum/2
  Sum/1 -> [P_load]
  EMS_Input_Conditioning/1(Ppv_ems) -> [P_pv]
  [P_pv] -> Sum1/1
  [P_grid_import] -> Sum1/2
  Sum2/1 -> [Pbat_ff]
  [P_load] -> Sum2/1
  Sum1/1 -> Sum2/2
  [P_pv] -> Sum3/1
  [P_load] -> Sum3/4
  EMS_Input_Conditioning/6(Pbat_ems) -> [Pbat_ems]
  [Pbat_ems] -> Sum3/2
  [P_grid_import] -> Sum3/3
  Sum3/1 -> [P_balance]

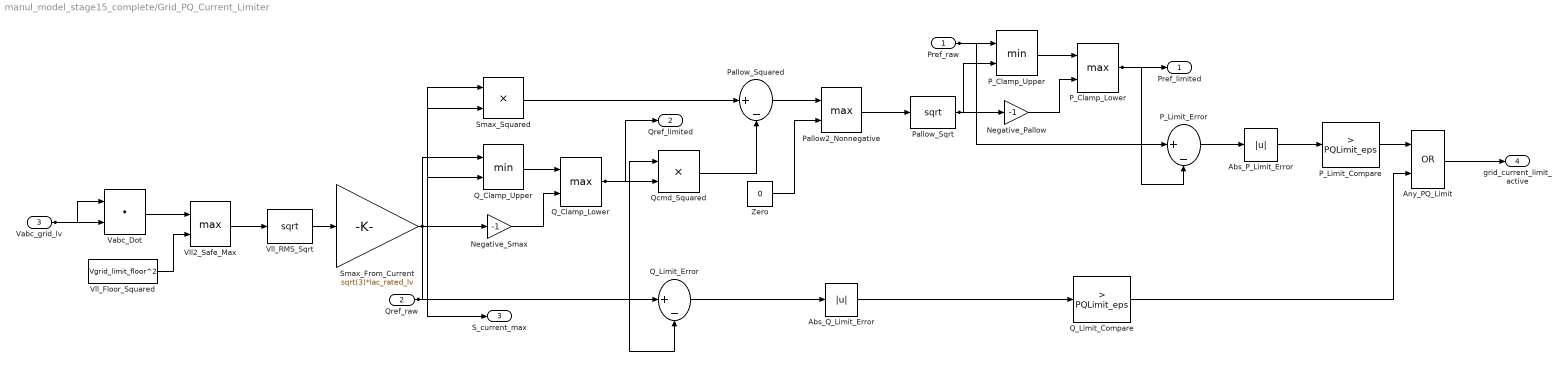
== system manul_model_stage15_complete/Grid_PQ_Current_Limiter ==
  Pref_raw : Inport
  Qref_raw : Inport  Port=2
  Vabc_grid_lv : Inport  Port=3
  Abs_P_Limit_Error : Abs  SaturateOnIntegerOverflow=off
  Abs_Q_Limit_Error : Abs  SaturateOnIntegerOverflow=off
  Any_PQ_Limit : Logic  Operator=OR  AllPortsSameDT=off  OutDataTypeStr=boolean
  Negative_Pallow : Gain  Gain=-1
  Negative_Smax : Gain  Gain=-1
  P_Clamp_Lower : MinMax  Function=max  Inputs=2
  P_Clamp_Upper : MinMax  Inputs=2
  P_Limit_Compare : simulink/Logic and Bit Operations/Compare To Constant  relop=>  const=PQLimit_eps  OutDataTypeStr=boolean
  P_Limit_Error : Sum  Inputs=|+-
  Pallow2_Nonnegative : MinMax  Function=max  Inputs=2
  Pallow_Sqrt : Math  Operator=sqrt
  Pallow_Squared : Sum  Inputs=|+-
  Q_Clamp_Lower : MinMax  Function=max  Inputs=2
  Q_Clamp_Upper : MinMax  Inputs=2
  Q_Limit_Compare : simulink/Logic and Bit Operations/Compare To Constant  relop=>  const=PQLimit_eps  OutDataTypeStr=boolean
  Q_Limit_Error : Sum  Inputs=|+-
  Qcmd_Squared : Product  Inputs=**
  Smax_From_Current : Gain  Gain=sqrt(3)*Iac_rated_lv
  Smax_Squared : Product  Inputs=**
  Vabc_Dot : DotProduct  OutDataTypeStr=Inherit: Inherit via internal rule
  Vll2_Safe_Max : MinMax  Function=max  Inputs=2
  Vll_Floor_Squared : Constant  Value=Vgrid_limit_floor^2
  Vll_RMS_Sqrt : Math  Operator=sqrt
  Zero : Constant  Value=0
  Pref_limited : Outport
  Qref_limited : Outport  Port=2
  S_current_max : Outport  Port=3
  grid_current_limit_active : Outport  Port=4
  wires:
  Qref_raw/1 -> Q_Clamp_Upper/1, Q_Limit_Error/1
  Vabc_grid_lv/1 -> Vabc_Dot/1, Vabc_Dot/2
  Smax_Squared/1 -> Pallow_Squared/1
  Negative_Smax/1 -> Q_Clamp_Lower/2
  Smax_From_Current/1 -> S_current_max/1, Q_Clamp_Upper/2, Negative_Smax/1, Smax_Squared/1, Smax_Squared/2
  Vabc_Dot/1 -> Vll2_Safe_Max/1
  Vll_Floor_Squared/1 -> Vll2_Safe_Max/2
  Vll_RMS_Sqrt/1 -> Smax_From_Current/1
  Vll2_Safe_Max/1 -> Vll_RMS_Sqrt/1
  Q_Clamp_Upper/1 -> Q_Clamp_Lower/1
  Negative_Pallow/1 -> P_Clamp_Lower/2
  Qcmd_Squared/1 -> Pallow_Squared/2
  Q_Clamp_Lower/1 -> Q_Limit_Error/2, Qref_limited/1, Qcmd_Squared/1, Qcmd_Squared/2
  Q_Limit_Error/1 -> Abs_Q_Limit_Error/1
  Pallow_Squared/1 -> Pallow2_Nonnegative/1
  Zero/1 -> Pallow2_Nonnegative/2
  Pallow2_Nonnegative/1 -> Pallow_Sqrt/1
  Abs_Q_Limit_Error/1 -> Q_Limit_Compare/1
  Pref_raw/1 -> P_Limit_Error/1, P_Clamp_Upper/1
  Pallow_Sqrt/1 -> P_Clamp_Upper/2, Negative_Pallow/1
  P_Clamp_Upper/1 -> P_Clamp_Lower/1
  P_Clamp_Lower/1 -> P_Limit_Error/2, Pref_limited/1
  Q_Limit_Compare/1 -> Any_PQ_Limit/2
  P_Limit_Error/1 -> Abs_P_Limit_Error/1
  Abs_P_Limit_Error/1 -> P_Limit_Compare/1
  P_Limit_Compare/1 -> Any_PQ_Limit/1
  Any_PQ_Limit/1 -> grid_current_limit_active/1

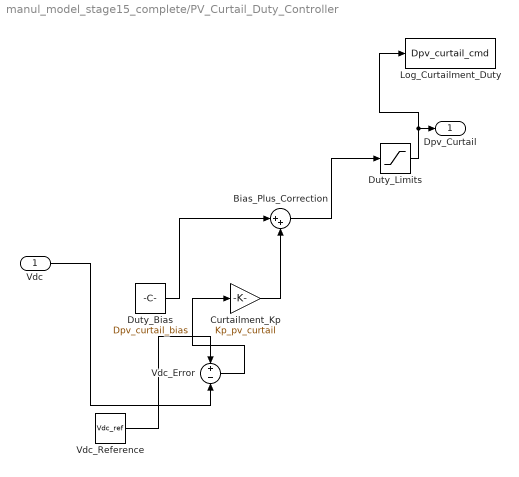
== system manul_model_stage15_complete/PV_Curtail_Duty_Controller ==
  Vdc : Inport
  Bias_Plus_Correction : Sum  Inputs=|++
  Curtailment_Kp : Gain  Gain=Kp_pv_curtail
  Duty_Bias : Constant  Value=Dpv_curtail_bias
  Duty_Limits : Saturate  UpperLimit=Dpv_max  LowerLimit=Dpv_min
  Log_Curtailment_Duty : ToWorkspace  VariableName=Dpv_curtail_cmd  SaveFormat=Timeseries
      settings: Decimation=20
  Vdc_Error : Sum  Inputs=+-
  Vdc_Reference : Constant  Value=Vdc_ref
  Dpv_Curtail : Outport
  wires:
  Vdc_Reference/1 -> Vdc_Error/1
  Vdc/1 -> Vdc_Error/2
  Vdc_Error/1 -> Curtailment_Kp/1
  Curtailment_Kp/1 -> Bias_Plus_Correction/2
  Duty_Bias/1 -> Bias_Plus_Correction/1
  Bias_Plus_Correction/1 -> Duty_Limits/1
  Duty_Limits/1 -> Log_Curtailment_Duty/1, Dpv_Curtail/1

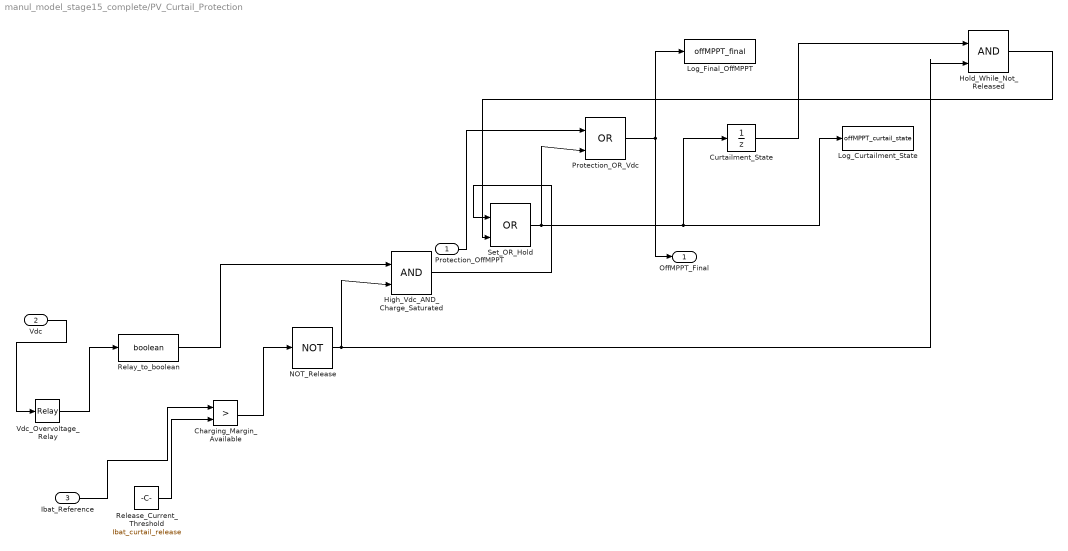
== system manul_model_stage15_complete/PV_Curtail_Protection ==
  Protection_OffMPPT : Inport
  Vdc : Inport  Port=2
  Ibat_Reference : Inport  Port=3
  Charging_Margin_Available : RelationalOperator  Operator=>
  Curtailment_State : UnitDelay  SampleTime=Ts_bat_ctrl
  High_Vdc_AND_Charge_Saturated : Logic  IconShape=distinctive
  Hold_While_Not_Released : Logic  IconShape=distinctive
  Log_Curtailment_State : ToWorkspace  VariableName=offMPPT_curtail_state  SaveFormat=Timeseries
      settings: Decimation=20
  Log_Final_OffMPPT : ToWorkspace  VariableName=offMPPT_final  SaveFormat=Timeseries
      settings: Decimation=20
  NOT_Release : Logic  Operator=NOT  Inputs=1  IconShape=distinctive
  Protection_OR_Vdc : Logic  Operator=OR  IconShape=distinctive
  Relay_to_boolean : DataTypeConversion  OutDataTypeStr=boolean
  Release_Current_Threshold : Constant  Value=Ibat_curtail_release
  Set_OR_Hold : Logic  Operator=OR  IconShape=distinctive
  Vdc_Overvoltage_Relay : Relay  OnSwitchValue=Vdc_curtail_on  OffSwitchValue=Vdc_curtail_off  OutDataTypeStr=double
  OffMPPT_Final : Outport
  wires:
  Ibat_Reference/1 -> Charging_Margin_Available/1
  Release_Current_Threshold/1 -> Charging_Margin_Available/2
  Charging_Margin_Available/1 -> NOT_Release/1
  NOT_Release/1 -> High_Vdc_AND_Charge_Saturated/2, Hold_While_Not_Released/2
  Curtailment_State/1 -> Hold_While_Not_Released/1
  Hold_While_Not_Released/1 -> Set_OR_Hold/2
  High_Vdc_AND_Charge_Saturated/1 -> Set_OR_Hold/1
  Set_OR_Hold/1 -> Log_Curtailment_State/1, Curtailment_State/1, Protection_OR_Vdc/2
  Relay_to_boolean/1 -> High_Vdc_AND_Charge_Saturated/1
  Protection_OffMPPT/1 -> Protection_OR_Vdc/1
  Vdc/1 -> Vdc_Overvoltage_Relay/1
  Vdc_Overvoltage_Relay/1 -> Relay_to_boolean/1
  Protection_OR_Vdc/1 -> OffMPPT_Final/1, Log_Final_OffMPPT/1

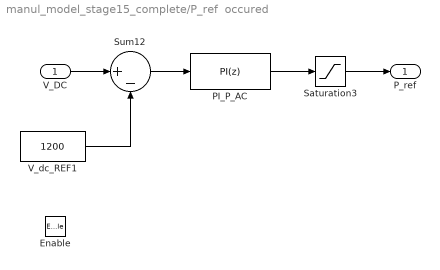
== system manul_model_stage15_complete/P_ref  occured ==
  V_DC : Inport
  Enable : EnablePort
  PI_P_AC : slpidlib/PID Controller  Controller=PI  Form=Parallel  TimeDomain=Discrete-time  UseExternalTs=off  SampleTime=Ts_mpc  IntegratorMethod=Forward Euler  FilterMethod=Forward Euler  ControllerParametersSource=internal  P=Kp_dc  I=Ki_dc  UseKiTs=off  D=0  UseExternalDerivativeSource=off  N=100  UseFilter=on  TunerSelectOption=Transfer Function Based (PID Tuner App)  InitialConditionSource=internal  InitialConditionForIntegrator=0  InitialConditionForFilter=0  DifferentiatorICPrevScaledInput=0  ExternalReset=none  TrackingMode=off  Kt=Kt_dc  LimitOutput=on  SatLimitsSource=internal  UpperSaturationLimit=Pref_max  LowerSaturationLimit=Pref_min  LinearizeAsGain=off  AntiWindupMode=clamping  Kb=1  LimitIntegrator=off  UpperIntegratorSaturationLimit=inf  LowerIntegratorSaturationLimit=-inf  POutMin=[]  POutMax=[]  IOutMin=[]  IOutMax=[]  DOutMin=[]  DOutMax=[]  NOutMin=[]  NOutMax=[]  SumOutMin=[]  SumOutMax=[]  SaturationOutMin=[]  SaturationOutMax=[]  PParamMin=[]  PParamMax=[]  IParamMin=[]  IParamMax=[]  DParamMin=[]  DParamMax=[]  NParamMin=[]  NParamMax=[]  KbParamMin=[]  KbParamMax=[]  KtParamMin=[]  KtParamMax=[]  KbOutMin=[]  KbOutMax=[]  KtOutMin=[]  KtOutMax=[]  IntegratorOutMin=[]  IntegratorOutMax=[]  FilterOutMin=[]  FilterOutMax=[]  SumI1OutMin=[]  SumI1OutMax=[]  SumI2OutMin=[]  SumI2OutMax=[]  SumI3OutMin=[]  SumI3OutMax=[]  SumI4OutMin=[]  SumI4OutMax=[]  SumDOutMin=[]  SumDOutMax=[]  DifferentiatorOutMin=[]  DifferentiatorOutMax=[]  FilterDiffOutCoefMin=[]  FilterDiffOutCoefMax=[]  ReciprocalOutMin=[]  ReciprocalOutMax=[]  SumDenOutMin=[]  SumDenOutMax=[]  SumNumOutMin=[]  SumNumOutMax=[]  DivideOutMin=[]  DivideOutMax=[]  UdiffTsProdOutMin=[]  UdiffTsProdOutMax=[]  NTsProdOutMin=[]  NTsProdOutMax=[]  UintegralTsProdOutMin=[]  UintegralTsProdOutMax=[]  UngainTsProdOutMin=[]  UngainTsProdOutMax=[]  ClampingZeroOutDataTypeStr=Inherit: Inherit via back propagation  ClampingZeroOutMin=[]  ClampingZeroOutMax=[]  FilterDenConstantOutDataTypeStr=Inherit: Inherit via back propagation  FilterDenConstantOutMin=[]  FilterDenConstantOutMax=[]  PCopyOutDataTypeStr=Inherit: Inherit via back propagation  PCopyOutMin=[]  PCopyOutMax=[]  NCopyOutDataTypeStr=Inherit: Inherit via back propagation  NCopyOutMin=[]  NCopyOutMax=[]  IntegratorContinuousStateAttributes=''  IntegratorStateMustResolveToSignalObject=off  IntegratorRTWStateStorageClass=Auto  FilterContinuousStateAttributes=''  FilterStateMustResolveToSignalObject=off  FilterRTWStateStorageClass=Auto  ParallelPVariant=InternalParameters  IdealPVariant=Disabled  IVariant=InternalParameters  DVariant=Disabled  IntegratorVariant=Discrete  SatVariant=Enabled  AWVariant=DiscClampingParallel  PCopyVariant=Disabled  TRVariant=Disabled  FdbkBlocksVariant=Forward  IdealPFdbkVariant=Disabled  SatFdbkVariant=Disabled  DerivativeFilterVariant=Disabled  NVariant=Disabled  NCopyVariant=Disabled_SignalSpec  FilterICVariant=Disabled  IntegratorICVariant=InternalICs  ExternalResetVariant=Disabled  TRSumVariant=Passthrough  SumFdbkVariant=Disabled  SumVariant=Sum_PI  TsampFilterVariant=InternalTs  TsampNgainVariant=Passthrough  TsampIntegralVariant=Disabled_SignalSpec  ExternalSaturationOutDataTypeStr=Inherit: Same as second input  DerivativeSourceVariant=Disabled  PreIntVariant=InternalPreInt
      settings: LibrarySourceBlock=simulink/Discrete/Discrete PID Controller
  Saturation3 : Saturate  UpperLimit=Pref_max  LowerLimit=Pref_min
  Sum12 : Sum  Inputs=|+-
  V_dc_REF1 : Constant  Value=1200
  P_ref : Outport
  wires:
  Sum12/1 -> PI_P_AC/1
  PI_P_AC/1 -> Saturation3/1
  Saturation3/1 -> P_ref/1
  V_DC/1 -> Sum12/1
  V_dc_REF1/1 -> Sum12/2

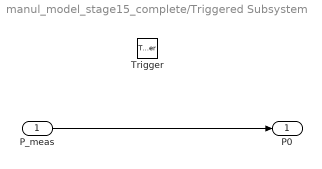
== system manul_model_stage15_complete/Triggered Subsystem ==
  P_meas : Inport
  Trigger : TriggerPort  VariantControl=(inherit)
  P0 : Outport
  wires:
  P_meas/1 -> P0/1

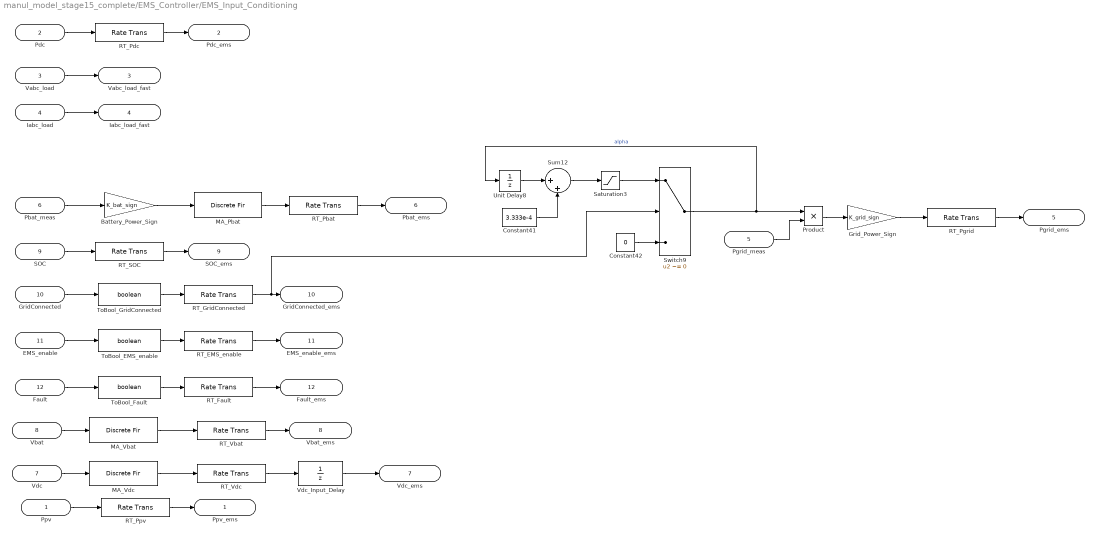
== system manul_model_stage15_complete/EMS_Controller/EMS_Input_Conditioning ==
  Ppv : Inport  OutDataTypeStr=double  PortDimensions=1
  Pdc : Inport  Port=2  OutDataTypeStr=double  PortDimensions=1
  Vabc_load : Inport  Port=3  OutDataTypeStr=double  PortDimensions=3
  Iabc_load : Inport  Port=4  OutDataTypeStr=double  PortDimensions=3
  Pgrid_meas : Inport  Port=5  OutDataTypeStr=double  PortDimensions=1
  Pbat_meas : Inport  Port=6  OutDataTypeStr=double  PortDimensions=1
  Vdc : Inport  Port=7  OutDataTypeStr=double  PortDimensions=1
  Vbat : Inport  Port=8  OutDataTypeStr=double  PortDimensions=1
  SOC : Inport  Port=9  OutDataTypeStr=double  PortDimensions=1
  GridConnected : Inport  Port=10  OutDataTypeStr=boolean  PortDimensions=1
  EMS_enable : Inport  Port=11  OutDataTypeStr=boolean  PortDimensions=1
  Fault : Inport  Port=12  OutDataTypeStr=boolean  PortDimensions=1
  Battery_Power_Sign : Gain  Gain=K_bat_sign
  Constant41 : Constant  Value=3.333e-4
  Constant42 : Constant  Value=0
  Grid_Power_Sign : Gain  Gain=K_grid_sign
  MA_Pbat : DiscreteFir  LoadFcn=dspblkCoreblockFVToolHelper(gcbh,'load');  Coefficients=ones(1,N_ems_fast_avg)/N_ems_fast_avg  SampleTime=Ts_power
      settings: CopyFcn=dspblkCoreblockFVToolHelper(gcbh,'copy');  DeleteFcn=dspblkCoreblockFVToolHelper(gcbh,'close');  ModelCloseFcn=dspblkCoreblockFVToolHelper(gcbh,'close');  PreSaveFcn=dspblkCoreblockFVToolHelper(gcbh,'presave');  PostSaveFcn=dspblkCoreblockFVToolHelper(gcbh,'postsave');  CloseFcn=dspblkCoreblockFVToolHelper(gcbh,'close');
  MA_Vbat : DiscreteFir  Coefficients=ones(1,N_ems_fast_avg)/N_ems_fast_avg  InitialStates=V_bat_nom  SampleTime=Ts_power
  MA_Vdc : DiscreteFir  Coefficients=ones(1,N_ems_fast_avg)/N_ems_fast_avg  InitialStates=Vdc_ref  SampleTime=Ts_power
  Product : Product
  RT_EMS_enable : RateTransition  OutPortSampleTime=Ts_ems
  RT_Fault : RateTransition  OutPortSampleTime=Ts_ems
  RT_GridConnected : RateTransition  OutPortSampleTime=Ts_ems
  RT_Pbat : RateTransition  OutPortSampleTime=Ts_ems
  RT_Pdc : RateTransition  OutPortSampleTime=Ts_ems
  RT_Pgrid : RateTransition  OutPortSampleTime=Ts_ems
  RT_Ppv : RateTransition  OutPortSampleTime=Ts_ems
  RT_SOC : RateTransition  OutPortSampleTime=Ts_ems
  RT_Vbat : RateTransition  OutPortSampleTime=Ts_ems
  RT_Vdc : RateTransition  OutPortSampleTime=Ts_ems
  Saturation3 : Saturate  UpperLimit=1  LowerLimit=0
  Sum12 : Sum  Inputs=|++
  Switch9 : Switch  Criteria=u2 ~= 0  SaturateOnIntegerOverflow=off  InputSameDT=off
  ToBool_EMS_enable : DataTypeConversion  OutDataTypeStr=boolean
  ToBool_Fault : DataTypeConversion  OutDataTypeStr=boolean
  ToBool_GridConnected : DataTypeConversion  OutDataTypeStr=boolean
  Unit Delay8 : UnitDelay  SampleTime=-1  HasFrameUpgradeWarning=on
  Vdc_Input_Delay : UnitDelay  InitialCondition=Vdc_ref  SampleTime=Ts_ems
  Ppv_ems : Outport  OutDataTypeStr=double  PortDimensions=1
  Pdc_ems : Outport  Port=2  OutDataTypeStr=double  PortDimensions=1
  Vabc_load_fast : Outport  Port=3  OutDataTypeStr=double  PortDimensions=3
  Iabc_load_fast : Outport  Port=4  OutDataTypeStr=double  PortDimensions=3
  Pgrid_ems : Outport  Port=5  OutDataTypeStr=double  PortDimensions=1
  Pbat_ems : Outport  Port=6  OutDataTypeStr=double  PortDimensions=1
  Vdc_ems : Outport  Port=7  OutDataTypeStr=double  PortDimensions=1
  Vbat_ems : Outport  Port=8  OutDataTypeStr=double  PortDimensions=1
  SOC_ems : Outport  Port=9  OutDataTypeStr=double  PortDimensions=1
  GridConnected_ems : Outport  Port=10  OutDataTypeStr=boolean  PortDimensions=1
  EMS_enable_ems : Outport  Port=11  OutDataTypeStr=boolean  PortDimensions=1
  Fault_ems : Outport  Port=12  OutDataTypeStr=boolean  PortDimensions=1
  wires:
  RT_Fault/1 -> Fault_ems/1
  ToBool_Fault/1 -> RT_Fault/1
  Fault/1 -> ToBool_Fault/1
  RT_EMS_enable/1 -> EMS_enable_ems/1
  ToBool_EMS_enable/1 -> RT_EMS_enable/1
  EMS_enable/1 -> ToBool_EMS_enable/1
  ToBool_GridConnected/1 -> RT_GridConnected/1
  GridConnected/1 -> ToBool_GridConnected/1
  RT_SOC/1 -> SOC_ems/1
  SOC/1 -> RT_SOC/1
  RT_Vbat/1 -> Vbat_ems/1
  Vdc_Input_Delay/1 -> Vdc_ems/1
  RT_Vdc/1 -> Vdc_Input_Delay/1
  RT_Pbat/1 -> Pbat_ems/1
  Pbat_meas/1 -> Battery_Power_Sign/1
  RT_Pgrid/1 -> Pgrid_ems/1
  Grid_Power_Sign/1 -> RT_Pgrid/1
  Iabc_load/1 -> Iabc_load_fast/1
  Vabc_load/1 -> Vabc_load_fast/1
  RT_Pdc/1 -> Pdc_ems/1
  Pdc/1 -> RT_Pdc/1
  RT_Ppv/1 -> Ppv_ems/1
  Ppv/1 -> RT_Ppv/1
  Battery_Power_Sign/1 -> MA_Pbat/1
  MA_Pbat/1 -> RT_Pbat/1
  Vdc/1 -> MA_Vdc/1
  MA_Vdc/1 -> RT_Vdc/1
  Vbat/1 -> MA_Vbat/1
  MA_Vbat/1 -> RT_Vbat/1
  RT_GridConnected/1 -> Switch9/2, GridConnected_ems/1
  Unit Delay8/1 -> Sum12/1
  Sum12/1 -> Saturation3/1
  Constant41/1 -> Sum12/2
  Saturation3/1 -> Switch9/1
  Constant42/1 -> Switch9/3
  Switch9/1 -> Product/1, Unit Delay8/1  "alpha"
  Pgrid_meas/1 -> Product/2
  Product/1 -> Grid_Power_Sign/1

== matlab function manul_model_stage15_complete/MATLAB Function2 ==
  data: Vdc input; gates output; Vg_ab input; P input; Q input; Pref input; Qref input; Ts input; Lf input; Rf input; omega input; Pbase input; Qbase input; lambda_sw input; previousState input; stateIndex output; Jmin output
function [gates,stateIndex,Jmin] = pvess_mppc_block( ...
    Vdc,Vg_ab,P,Q,Pref,Qref,Ts,Lf,Rf,omega,Pbase,Qbase, ...
    lambda_sw,previousState)
%PVESS_MPPC_BLOCK Code for the grid-connected MATLAB Function block.
% Copy this whole function into a MATLAB Function block, or call it from
% that block. The equations follow the paper's P/Q predictive model.
%
% IMPORTANT SIGN CONVENTION:
% P,Q and the measured current must use one consistent direction.
% SIGN CONVENTION:
% Filter current If is positive from inverter toward grid.
% Positive active power P means power exported from inverter/microgrid
% toward the grid. 
% If the Current Measurement arrow points from
% converter toward grid, multiply that current by -1 before P/Q calculation.

states = [0 0 0; ...
          1 0 0; ...
          1 1 0; ...
          0 1 0; ...
          0 1 1; ...
          0 0 1; ...
          1 0 1; ...
          1 1 1];

Jmin = inf;
stateIndex = 1;
previousState = previousState(:).';
Vg2 = Vg_ab(1)^2 + Vg_ab(2)^2;

for k = 1:8
    s = states(k,:);
    Vi_alpha = (2/3)*Vdc*(s(1)-0.5*s(2)-0.5*s(3));
    Vi_beta  = (sqrt(3)/3)*Vdc*(s(2)-s(3));

    % real/imaginary parts of Vg*conj(Vi).
    realTerm = Vg_ab(1)*Vi_alpha + Vg_ab(2)*Vi_beta;
    imagTerm = Vg_ab(2)*Vi_alpha - Vg_ab(1)*Vi_beta;

    % Paper active/reactive power one-step prediction.
    Ppred = P + Ts*(-Rf/Lf*P - omega*Q ...
        + 3/(2*Lf)*(realTerm - Vg2));
    Qpred = Q + Ts*( omega*P - Rf/Lf*Q ...
        + 3/(2*Lf)*imagTerm);

    Jpq = ((Pref-Ppred)/Pbase)^2 + ((Qref-Qpred)/Qbase)^2;
    Jsw = lambda_sw*sum(abs(s-previousState));
    J = Jpq + Jsw;

    if J < Jmin
        Jmin = J;
        stateIndex = k;
    end
end

s = states(stateIndex,:);
gates = [s(1);1-s(1);s(2);1-s(2);s(3);1-s(3)];
end
